simulink library "mfeval_STI_LIB"  (R2017b)
settings: Solver=ode45  StartTime=0.0  StopTime=10.0  RelTol=1e-3
undefined symbols (not defined in the file or in its folder): parameterStruct, userDynamics
libraries: mfeval_LIB x3, mfeval_CPI_LIB x1
settings Model: Creator=MFURLANT  LastModifiedBy=MFURLANT
settings DataIOCC: SaveFormat=StructureWithTime
settings OptimizationCC: LifeSpan=inf
settings DebuggingCC: SFExecutionAtInitializationDiag=none
settings HardwareCC: ProdBitPerSizeT=32  ProdBitPerPtrDiffT=32  ProdWordSize=32  ProdHWDeviceType=Specified
settings CodeAppCC: StateflowObjectComments=on
settings GRTTargetCC: TargetLangStandard=C89/C90 (ANSI)

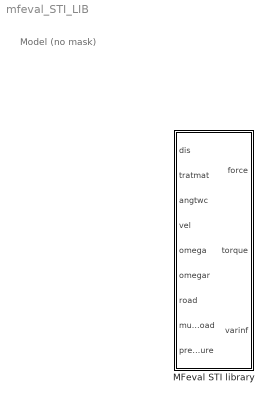
== system mfeval_STI_LIB ==
  note: Model (no mask)
  MFeval STI library : Subsystem

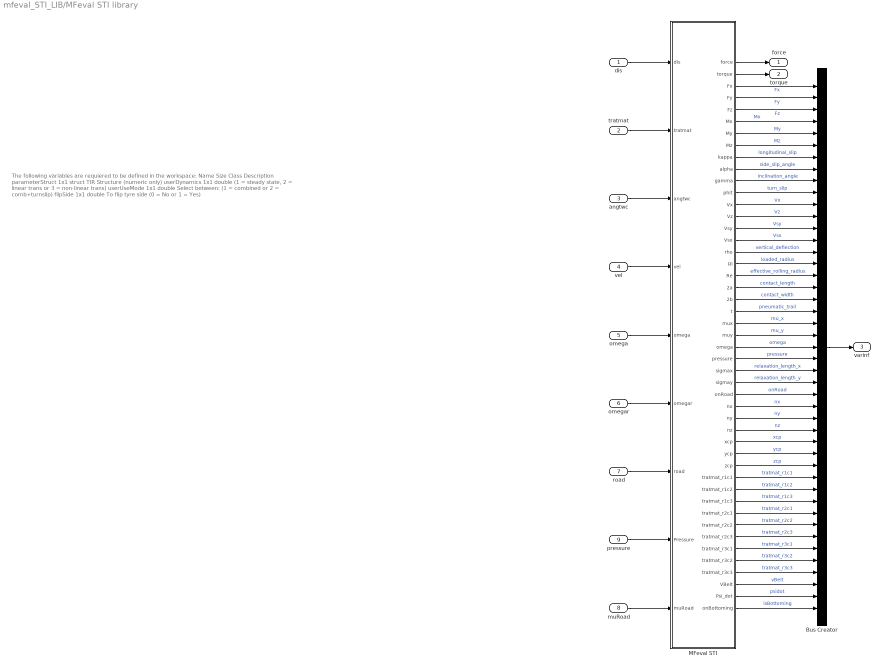
== system mfeval_STI_LIB/MFeval STI library ==
  note: The following variables are requiered to be defined in the workspace:
      |
      | Name
      | Size
      | Class
      | Description
      |
      | parameterStruct
      | 1x1
      | struct
      | TIR Structure (numeric only)
      |
      | userDynamics
      | 1x1
      | double
      | (1 = steady state, 2 = linear trans or 3 = non-linear trans)
      |
      | userUseMode
      | 1x1
      | double
      | Select between: (1 = combined or 2 = comb+turnslip)
      |
      | flipSide
      | 1x1
      | double
      | To flip tyre side (0 = No or 1 = Yes)
  dis : Inport
  tratmat : Inport  Port=2
  angtwc : Inport  Port=3
  vel : Inport  Port=4
  omega : Inport  Port=5
  omegar : Inport  Port=6
  road : Inport  Port=7
  muRoad : Inport  Port=8
  pressure : Inport  Port=9
  Bus Creator : BusCreator  Inputs=45
  MFeval STI : Subsystem
  force : Outport
  torque : Outport  Port=2
  varinf : Outport  Port=3
  wires:
  MFeval STI/7(My) -> Bus Creator/5  "My"
  MFeval STI/17(rho) -> Bus Creator/15  "vertical_deflection"
  MFeval STI/9(kappa) -> Bus Creator/7  "longitudinal_slip"
  MFeval STI/13(Vx) -> Bus Creator/11  "Vx"
  MFeval STI/8(Mz) -> Bus Creator/6  "Mz"
  MFeval STI/14(Vz) -> Bus Creator/12  "Vz"
  MFeval STI/10(alpha) -> Bus Creator/8  "side_slip_angle"
  MFeval STI/16(Vsx) -> Bus Creator/14  "Vsx"
  MFeval STI/1(force) -> force/1
  MFeval STI/2(torque) -> torque/1
  Bus Creator/1 -> varinf/1
  MFeval STI/3(Fx) -> Bus Creator/1  "Fx"
  MFeval STI/4(Fy) -> Bus Creator/2  "Fy"
  MFeval STI/5(Fz) -> Bus Creator/3  "Fz"
  MFeval STI/6(Mx) -> Bus Creator/4  "Mx"
  MFeval STI/19(Re) -> Bus Creator/17  "effective_rolling_radius"
  MFeval STI/15(Vsy) -> Bus Creator/13  "Vsy"
  MFeval STI/18(Rl) -> Bus Creator/16  "loaded_radius"
  MFeval STI/11(gamma) -> Bus Creator/9  "inclination_angle"
  MFeval STI/20(2a) -> Bus Creator/18  "contact_length"
  MFeval STI/27(sigmax) -> Bus Creator/25  "relaxation_length_x"
  MFeval STI/28(sigmay) -> Bus Creator/26  "relaxation_length_y"
  MFeval STI/23(mux) -> Bus Creator/21  "mu_x"
  MFeval STI/22(t) -> Bus Creator/20  "pneumatic_trail"
  MFeval STI/26(pressure) -> Bus Creator/24  "pressure"
  MFeval STI/12(phit) -> Bus Creator/10  "turn_slip"
  MFeval STI/24(muy) -> Bus Creator/22  "mu_y"
  MFeval STI/25("omega ") -> Bus Creator/23  "omega"
  MFeval STI/21(2b) -> Bus Creator/19  "contact_width"
  MFeval STI/29(onRoad) -> Bus Creator/27  "onRoad"
  MFeval STI/30(nx) -> Bus Creator/28  "nx"
  MFeval STI/31(ny) -> Bus Creator/29  "ny"
  MFeval STI/32(nz) -> Bus Creator/30  "nz"
  MFeval STI/33(xcp) -> Bus Creator/31  "xcp"
  MFeval STI/34(ycp) -> Bus Creator/32  "ycp"
  MFeval STI/35(zcp) -> Bus Creator/33  "zcp"
  MFeval STI/36(tratmat_r1c1) -> Bus Creator/34  "tratmat_r1c1"
  MFeval STI/37(tratmat_r1c2) -> Bus Creator/35  "tratmat_r1c2"
  MFeval STI/38(tratmat_r1c3) -> Bus Creator/36  "tratmat_r1c3"
  MFeval STI/39(tratmat_r2c1) -> Bus Creator/37  "tratmat_r2c1"
  MFeval STI/40(tratmat_r2c2) -> Bus Creator/38  "tratmat_r2c2"
  MFeval STI/41(tratmat_r2c3) -> Bus Creator/39  "tratmat_r2c3"
  MFeval STI/42(tratmat_r3c1) -> Bus Creator/40  "tratmat_r3c1"
  MFeval STI/43(tratmat_r3c2) -> Bus Creator/41  "tratmat_r3c2"
  MFeval STI/44(tratmat_r3c3) -> Bus Creator/42  "tratmat_r3c3"
  MFeval STI/45(VBelt) -> Bus Creator/43  "vBelt"
  MFeval STI/46(Psi_dot) -> Bus Creator/44  "psidot"
  muRoad/1 -> MFeval STI/9(muRoad)
  road/1 -> MFeval STI/7(road)
  omegar/1 -> MFeval STI/6(omegar)
  omega/1 -> MFeval STI/5(omega)
  vel/1 -> MFeval STI/4(vel)
  angtwc/1 -> MFeval STI/3(angtwc)
  tratmat/1 -> MFeval STI/2(tratmat)
  dis/1 -> MFeval STI/1(dis)
  pressure/1 -> MFeval STI/8(Pressure)
  MFeval STI/47(onBottoming) -> Bus Creator/45  "isBottoming"

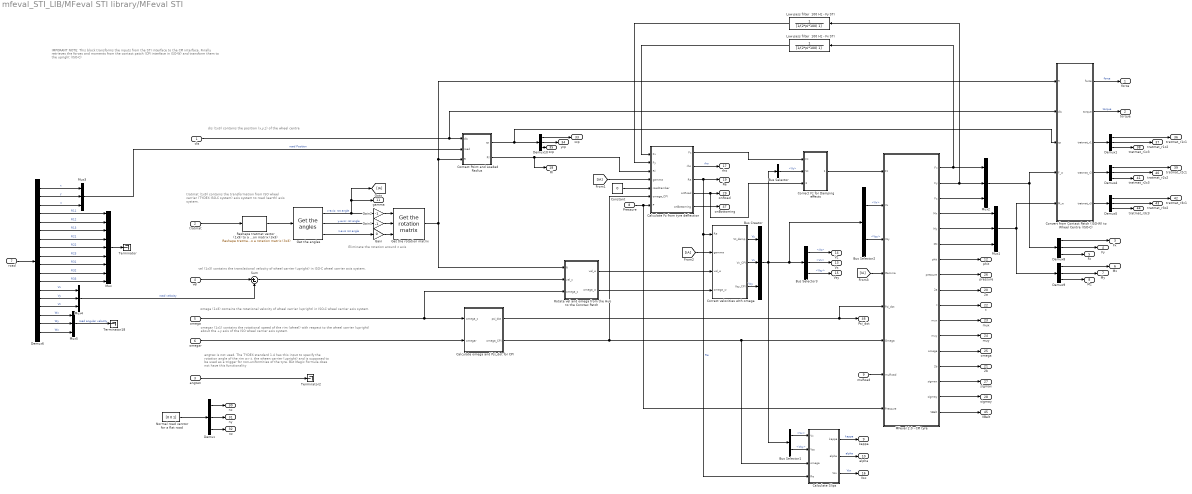
== system mfeval_STI_LIB/MFeval STI library/MFeval STI ==
  note: omegar (1x1) contains the rotational speed of the rim (wheel) with respect to the wheel carrier (upright) about the +y axis of the ISO wheel carrier axis system.
  note: omega (1x3) contains the rotational velocity of wheel carrier (upright) in ISO-C wheel carrier axis system.
  note: tratmat (1x9) contains the transformation from ISO wheel carrier (TYDEX ISO-C system) axis system to road (earth) axis system.
  note: vel (1x3) contains the translational velocity of wheel carrier (upright) in ISO-C wheel carrier axis system.
  note: IMPORANT NOTE:
      |
      | This block transforms the inputs from the STI interface to the CPI interface.
      | Finally retrieves the forces and moments from the contact patch (CPI interface in ISO-W) and transform them to the upright (ISO-C)
  note: angtwc is not used.
      | The TYDEX standard 1.4 has this input to specify the rotation angle of the rim w.r.t. the wheen carrier (upright) and is supposed to be used as a trigger for non-uniformities of the tyre. But Magic Formula does not have this functionality
  note: dis (1x3) contains the position (x,y,z) of the wheel centre
  note: Eliminate the rotation around z axis
  dis : Inport
  tratmat : Inport  Port=2
  angtwc : Inport  Port=3
  vel : Inport  Port=4
  omega : Inport  Port=5
  omegar : Inport  Port=6
  road : Inport  Port=7
  Pressure : Inport  Port=8
  muRoad : Inport  Port=9
  Bus Creator : BusCreator  Inputs=3
  Bus Selector : BusSelector  OutputSignals=Vz
  Bus Selector1 : BusSelector  OutputSignals=Vx,Vsy
  Bus Selector2 : BusSelector  OutputSignals=Vx,Vsy
  Bus Selector3 : BusSelector  OutputSignals=Vz,Vx,Vsy
  Calculate Fz from tyre deflection : MATLAB Function  TreatAsAtomicUnit=on
  Calculate Slips : MATLAB Function  TreatAsAtomicUnit=on
  Calculate omega and Psi_dot for CPI : Subsystem
  Constant : Constant  Value=0
  Contact Point and Loaded Radius : MATLAB Function  TreatAsAtomicUnit=on
  Convert from Contact Patch (ISO-W) to Wheel Centre (ISO-C) : MATLAB Function  TreatAsAtomicUnit=on
  Correct Fz for Damping effects : Subsystem
  Correct velocities with omega : Subsystem
  Demux{,1,4..5,8..10} (7 alike) : Demux  Outputs=3
  Demux6 : Demux  Outputs=18
  Gain : Gain  Gain=0
  Gain1 : Gain  Gain=-1
  Gain2 : Gain  Gain=-1
  Get the angles : mfeval_LIB/Get the angles
      settings: SourceProductName=MFeval Library
  Get the rotation matrix : mfeval_LIB/Get the rotation matrix
      settings: SourceProductName=MFeval Library
  Low pass filter  100 Hz - Fx STI : TransferFcn  Denominator=[1/(2*pi*100) 1]
  Low pass filter  100 Hz - Fy STI : TransferFcn  Denominator=[1/(2*pi*100) 1]
  MFeval 2.0 - CPI tyre : Subsystem
  Mux : Mux  Inputs=9
  Mux{1..5} (5 alike) : Mux  Inputs=3
  Normal road verctor for a flat road : Constant  Value=[0 0 1]
  Reshape tratmat vector (1x9) to a rotation matrix (3x3) : mfeval_LIB/Reshape tratmat vector (1x9)  to a rotation matrix (3x3)
      settings: SourceProductName=MFeval Library
  Rotate vel and omega from the Hub to the Conctac Patch : Subsystem
  Sum : Sum  Inputs=|+-
  Terminator : Terminator
  Terminator18 : Terminator
  Terminator2 : Terminator
  force : Outport
  torque : Outport  Port=2
  Fx : Outport  Port=3
  Fy : Outport  Port=4
  Fz : Outport  Port=5
  Mx : Outport  Port=6
  My : Outport  Port=7
  Mz : Outport  Port=8
  kappa : Outport  Port=9
  alpha : Outport  Port=10
  gamma : Outport  Port=11
  phit : Outport  Port=12
  Vx : Outport  Port=13
  Vz : Outport  Port=14
  Vsy : Outport  Port=15
  Vsx : Outport  Port=16
  rho : Outport  Port=17
  Rl : Outport  Port=18
  Re : Outport  Port=19
  2a : Outport  Port=20
  2b : Outport  Port=21
  t : Outport  Port=22
  mux : Outport  Port=23
  muy : Outport  Port=24
  "omega " : Outport  Port=25
  pressure : Outport  Port=26
  sigmax : Outport  Port=27
  sigmay : Outport  Port=28
  onRoad : Outport  Port=29
  nx : Outport  Port=30
  ny : Outport  Port=31
  nz : Outport  Port=32
  xcp : Outport  Port=33
  ycp : Outport  Port=34
  zcp : Outport  Port=35
  tratmat_r1c1 : Outport  Port=36
  tratmat_r1c2 : Outport  Port=37
  tratmat_r1c3 : Outport  Port=38
  tratmat_r2c1 : Outport  Port=39
  tratmat_r2c2 : Outport  Port=40
  tratmat_r2c3 : Outport  Port=41
  tratmat_r3c1 : Outport  Port=42
  tratmat_r3c2 : Outport  Port=43
  tratmat_r3c3 : Outport  Port=44
  VBelt : Outport  Port=45
  Psi_dot : Outport  Port=46
  onBottoming : Outport  Port=47
  wires:
  Contact Point and Loaded Radius/2(Rl) -> Rl/1, Calculate Fz from tyre deflection/3(Rl)
  angtwc/1 -> Terminator2/1
  MFeval 2.0 - CPI tyre/1(Fx) -> Low pass filter  100 Hz - Fx STI/1, Mux2/1
  MFeval 2.0 - CPI tyre/2(Fy) -> Low pass filter  100 Hz - Fy STI/1, Mux2/2
  tratmat/1 -> Reshape tratmat vector (1x9) to a rotation matrix (3x3)/1
  MFeval 2.0 - CPI tyre/4(Mx) -> Mux1/1
  MFeval 2.0 - CPI tyre/5(My) -> Mux1/2
  Mux1/1 -> Convert from Contact Patch (ISO-W) to Wheel Centre (ISO-C)/5(M_w), Demux9/1
  Mux2/1 -> Convert from Contact Patch (ISO-W) to Wheel Centre (ISO-C)/4(F_w), Demux8/1
  MFeval 2.0 - CPI tyre/3("Fz ") -> Mux2/3
  Get the angles/3 -> Gain/1  "z-axis rot angle"
  Get the angles/2 -> Gain1/1  "y-axis: rot angle"
  Convert from Contact Patch (ISO-W) to Wheel Centre (ISO-C)/1(force) -> force/1  "force"
  Convert from Contact Patch (ISO-W) to Wheel Centre (ISO-C)/2(torque) -> torque/1  "torque"
  omegar/1 -> Calculate omega and Psi_dot for CPI/2(omegar)
  Calculate Fz from tyre deflection/2(rho) -> rho/1  "rho"
  Calculate omega and Psi_dot for CPI/2(omega_CPI) -> Calculate Fz from tyre deflection/6(omega_CPI), MFeval 2.0 - CPI tyre/6(Omega), Calculate Slips/3(omega)
  Sum/1 -> Rotate vel and omega from the Hub to the Conctac Patch/2(vel_c)
  Calculate Fz from tyre deflection/1(Fz) -> Correct Fz for Damping effects/1(Fz)
  MFeval 2.0 - CPI tyre/6(Mz) -> Mux1/3
  MFeval 2.0 - CPI tyre/7(phit) -> phit/1
  MFeval 2.0 - CPI tyre/8(pressure) -> pressure/1
  MFeval 2.0 - CPI tyre/9(2a) -> 2a/1
  MFeval 2.0 - CPI tyre/10(t) -> t/1
  MFeval 2.0 - CPI tyre/11(mux) -> mux/1
  MFeval 2.0 - CPI tyre/12(muy) -> muy/1
  MFeval 2.0 - CPI tyre/13(omega) -> "omega "/1
  MFeval 2.0 - CPI tyre/14(2b) -> 2b/1
  MFeval 2.0 - CPI tyre/15(sigmax) -> sigmax/1
  MFeval 2.0 - CPI tyre/16(sigmay) -> sigmay/1
  Rotate vel and omega from the Hub to the Conctac Patch/1(vel_w) -> Correct velocities with omega/3(vel_w)
  Rotate vel and omega from the Hub to the Conctac Patch/2(omega_w) -> Correct velocities with omega/4(omega_w)
  Calculate Slips/1(kappa) -> kappa/1  "kappa"
  Calculate Slips/2(alpha) -> alpha/1  "alpha"
  Calculate Slips/3(Vsx) -> Vsx/1  "Vsx"
  Calculate Fz from tyre deflection/3(Re) -> Calculate Slips/4(Re), Correct velocities with omega/1(Re), Re/1  "Re"
  Correct velocities with omega/1(Vz_damp) -> Bus Creator/1  "Vz"
  Correct velocities with omega/2(Vx_CPI) -> Bus Creator/2  "Vx"
  Correct velocities with omega/3(Vsy_CPI) -> Bus Creator/3  "Vsy"
  Bus Creator/1 -> Bus Selector1/1, Bus Selector2/1, Bus Selector3/1, Bus Selector/1
  Bus Selector/1 -> Correct Fz for Damping effects/2(Vz)  "<Vz>"
  Bus Selector1/1 -> Calculate Slips/1(Vx)  "<Vx>"
  Bus Selector1/2 -> Calculate Slips/2(Vsy)  "<Vsy>"
  Bus Selector2/1 -> MFeval 2.0 - CPI tyre/2(Vx)  "<Vx>"
  Bus Selector2/2 -> MFeval 2.0 - CPI tyre/3(Vsy)  "<Vsy>"
  Bus Selector3/3 -> Vsy/1  "<Vsy>"
  Bus Selector3/2 -> Vx/1  "<Vx>"
  Bus Selector3/1 -> Vz/1  "<Vz>"
  Low pass filter  100 Hz - Fy STI/1 -> Calculate Fz from tyre deflection/2(Fy)
  Low pass filter  100 Hz - Fx STI/1 -> Calculate Fz from tyre deflection/1(Fx)
  Demux10/1 -> xcp/1
  Demux10/2 -> ycp/1
  Demux10/3 -> zcp/1
  Convert from Contact Patch (ISO-W) to Wheel Centre (ISO-C)/3(tratmat_r1) -> Demux1/1
  Convert from Contact Patch (ISO-W) to Wheel Centre (ISO-C)/4(tratmat_r2) -> Demux4/1
  Convert from Contact Patch (ISO-W) to Wheel Centre (ISO-C)/5(tratmat_r3) -> Demux5/1
  Demux1/1 -> tratmat_r1c1/1
  Demux1/2 -> tratmat_r1c2/1
  Demux1/3 -> tratmat_r1c3/1
  Demux4/1 -> tratmat_r2c1/1
  Demux4/2 -> tratmat_r2c2/1
  Demux4/3 -> tratmat_r2c3/1
  Demux5/1 -> tratmat_r3c1/1
  Demux5/2 -> tratmat_r3c2/1
  Demux5/3 -> tratmat_r3c3/1
  MFeval 2.0 - CPI tyre/17(VBelt) -> VBelt/1
  road/1 -> Demux6/1
  Demux6/1 -> Mux3/1  "x"
  Demux6/2 -> Mux3/2  "y"
  Demux6/3 -> Mux3/3  "z"
  Demux6/4 -> Mux/1  "R11"
  Demux6/5 -> Mux/2  "R12"
  Demux6/6 -> Mux/3  "R13"
  Demux6/7 -> Mux/4  "R21"
  Demux6/8 -> Mux/5  "R22"
  Demux6/9 -> Mux/6  "R23"
  Demux6/10 -> Mux/7  "R31"
  Demux6/11 -> Mux/8  "R32"
  Demux6/12 -> Mux/9  "R33"
  Demux6/13 -> Mux4/1  "Vx"
  Demux6/14 -> Mux4/2  "Vy"
  Demux6/15 -> Mux4/3  "Vz"
  Demux6/16 -> Mux5/1  "Wx"
  Demux6/17 -> Mux5/2  "Wy"
  Demux6/18 -> Mux5/3  "Wz"
  Mux3/1 -> Contact Point and Loaded Radius/2(road)  "road Position"
  Mux4/1 -> Sum/2  "road velocity"
  Get the angles/1 -> gamma/1, [IA], Gain2/1  "x-axis: rot angle"
  Demux8/1 -> Fx/1
  Demux8/2 -> Fy/1
  Demux8/3 -> Fz/1
  Demux9/1 -> Mx/1
  Demux9/2 -> My/1
  Demux9/3 -> Mz/1
  Demux/2 -> ny/1
  Demux/3 -> nz/1
  Demux/1 -> nx/1
  Normal road verctor for a flat road/1 -> Demux/1
  Constant/1 -> Calculate Fz from tyre deflection/5(roadCamber)
  dis/1 -> Convert from Contact Patch (ISO-W) to Wheel Centre (ISO-C)/2(dis), Contact Point and Loaded Radius/1(dis)
  Mux5/1 -> Terminator18/1  "road angular velocity"
  vel/1 -> Sum/1
  muRoad/1 -> MFeval 2.0 - CPI tyre/7(muRoad)
  Get the rotation matrix/1 -> Convert from Contact Patch (ISO-W) to Wheel Centre (ISO-C)/1(R), Contact Point and Loaded Radius/3(R), Rotate vel and omega from the Hub to the Conctac Patch/1(R)
  [IA] -> Calculate Fz from tyre deflection/4(gamma)
  [IA] -> Correct velocities with omega/2(gamma)
  [IA] -> MFeval 2.0 - CPI tyre/4(Gamma)
  Calculate Fz from tyre deflection/4(onRoad) -> Correct Fz for Damping effects/3(onRoad), onRoad/1
  Correct Fz for Damping effects/1(Fz_CPI) -> MFeval 2.0 - CPI tyre/1(Fz)
  Pressure/1 -> MFeval 2.0 - CPI tyre/8(Pressure), Calculate Fz from tyre deflection/7(P)
  omega/1 -> Rotate vel and omega from the Hub to the Conctac Patch/3(omega_c), Calculate omega and Psi_dot for CPI/1(omega_c)
  Calculate omega and Psi_dot for CPI/1(psi_dot) -> MFeval 2.0 - CPI tyre/5(Psi_dot), Psi_dot/1
  Calculate Fz from tyre deflection/5(onBottoming) -> onBottoming/1
  Contact Point and Loaded Radius/1(cp) -> Convert from Contact Patch (ISO-W) to Wheel Centre (ISO-C)/3(cp), Demux10/1
  Mux/1 -> Terminator/1
  Gain/1 -> Get the rotation matrix/3
  Reshape tratmat vector (1x9) to a rotation matrix (3x3)/1 -> Get the angles/1
  Gain1/1 -> Get the rotation matrix/2
  Gain2/1 -> Get the rotation matrix/1

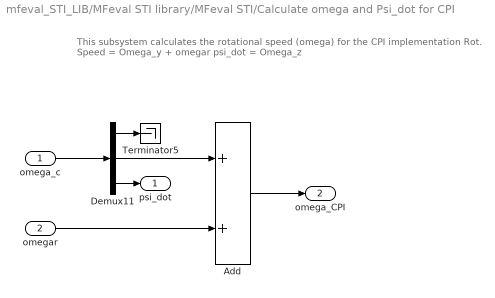
== system mfeval_STI_LIB/MFeval STI library/MFeval STI/Calculate omega and Psi_dot for CPI ==
  note: This subsystem calculates the rotational speed (omega) for the CPI implementation
      |
      | Rot. Speed = Omega_y + omegar
      | psi_dot = Omega_z
  omega_c : Inport
  omegar : Inport  Port=2
  Add : Sum
  Demux11 : Demux  Outputs=3
  Terminator5 : Terminator
  psi_dot : Outport
  omega_CPI : Outport  Port=2
  wires:
  Add/1 -> omega_CPI/1
  omega_c/1 -> Demux11/1
  omegar/1 -> Add/2
  Demux11/1 -> Terminator5/1
  Demux11/3 -> psi_dot/1
  Demux11/2 -> Add/1

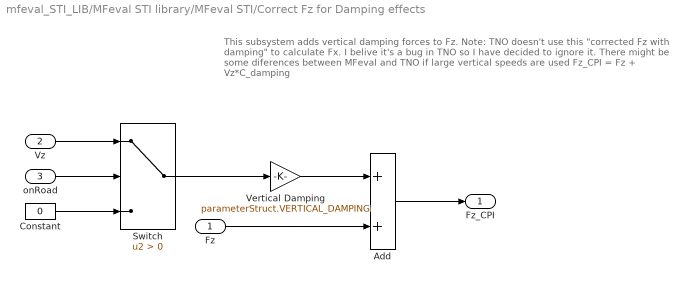
== system mfeval_STI_LIB/MFeval STI library/MFeval STI/Correct Fz for Damping effects ==
  note: This subsystem adds vertical damping forces to Fz.
      |
      | Note: TNO doesn't use this "corrected Fz with damping" to calculate Fx.
      | I belive it's a bug in TNO so I have decided to ignore it.
      | There might be some diferences between MFeval and TNO if large vertical speeds are used
      |
      |
      | Fz_CPI = Fz + Vz*C_damping
  Fz : Inport
  Vz : Inport  Port=2
  onRoad : Inport  Port=3
  Add : Sum
  Constant : Constant  Value=0
  Switch : Switch  Criteria=u2 > Threshold
  Vertical Damping : Gain  Gain=parameterStruct.VERTICAL_DAMPING
  Fz_CPI : Outport
  wires:
  Fz/1 -> Add/2
  Add/1 -> Fz_CPI/1
  Vz/1 -> Switch/1
  Vertical Damping/1 -> Add/1
  onRoad/1 -> Switch/2
  Constant/1 -> Switch/3
  Switch/1 -> Vertical Damping/1

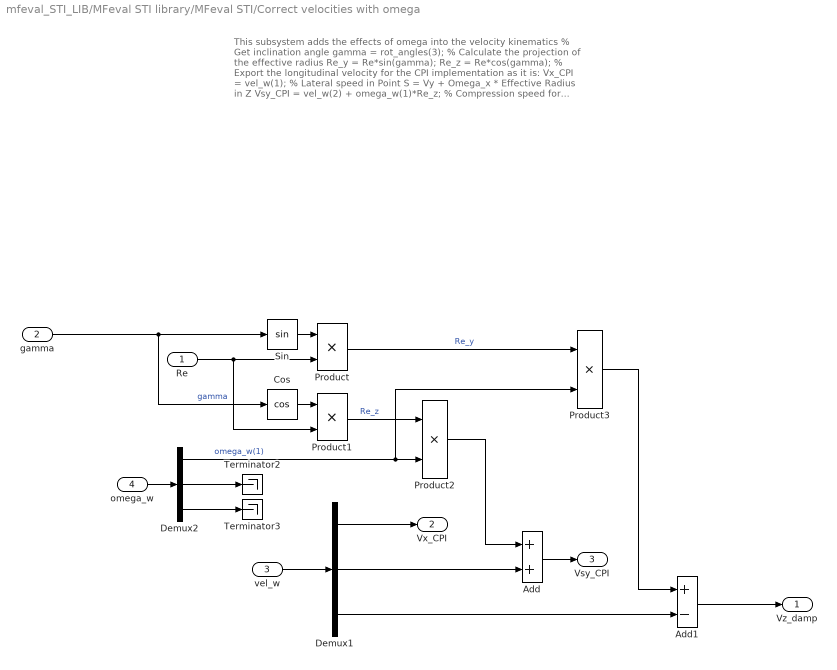
== system mfeval_STI_LIB/MFeval STI library/MFeval STI/Correct velocities with omega ==
  note: This subsystem adds the effects of omega into the velocity kinematics
      |
      | % Get inclination angle
      | gamma = rot_angles(3);
      |
      | % Calculate the projection of the effective radius
      | Re_y = Re*sin(gamma);
      | Re_z = Re*cos(gamma);
      |
      | % Export the longitudinal velocity for the CPI implementation as it is:
      | Vx_CPI = vel_w(1);
      |
      | % Lateral speed in Point S = Vy + Omega_x * Effective Radius in Z
      | Vsy_CPI = vel_w(2) + omega_w(1)*Re_z;
      |
      | % Compression speed for damping effects:
      | Vz_damp = vel_w(3) + omega_w(1)*Re_y;
  Re : Inport
  gamma : Inport  Port=2
  vel_w : Inport  Port=3
  omega_w : Inport  Port=4
  Add : Sum
  Add1 : Sum  Inputs=+-
  Cos : Trigonometry  Operator=cos
  Demux1 : Demux  Outputs=3
  Demux2 : Demux  Outputs=3
  Product{,1..3} (4 alike) : Product
  Sin : Trigonometry
  Terminator2 : Terminator
  Terminator3 : Terminator
  Vz_damp : Outport
  Vx_CPI : Outport  Port=2
  Vsy_CPI : Outport  Port=3
  wires:
  gamma/1 -> Sin/1, Cos/1  "gamma"
  Sin/1 -> Product/1
  Re/1 -> Product1/2, Product/2
  Cos/1 -> Product1/1
  Product/1 -> Product3/1  "Re_y"
  Product1/1 -> Product2/1  "Re_z"
  vel_w/1 -> Demux1/1
  Demux1/1 -> Vx_CPI/1
  Demux1/2 -> Add/2
  omega_w/1 -> Demux2/1
  Demux2/3 -> Terminator3/1
  Demux2/2 -> Terminator2/1
  Demux2/1 -> Product3/2, Product2/2  "omega_w(1)"
  Product2/1 -> Add/1
  Add/1 -> Vsy_CPI/1
  Product3/1 -> Add1/1
  Demux1/3 -> Add1/2
  Add1/1 -> Vz_damp/1

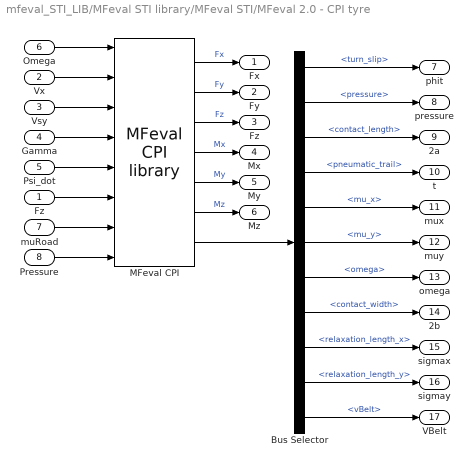
== system mfeval_STI_LIB/MFeval STI library/MFeval STI/MFeval 2.0 - CPI tyre ==
  Fz : Inport
  Vx : Inport  Port=2
  Vsy : Inport  Port=3
  Gamma : Inport  Port=4
  Psi_dot : Inport  Port=5
  Omega : Inport  Port=6
  muRoad : Inport  Port=7
  Pressure : Inport  Port=8
  Bus Selector : BusSelector  OutputSignals=turn_slip,pressure,contact_length,pneumatic_trail,mu_x,mu_y,omega,contact_width,relaxation_length_x,relaxation_length_y,vBelt
  MFeval CPI : mfeval_CPI_LIB/MFeval CPI library
  Fx : Outport
  Fy : Outport  Port=2
  "Fz " : Outport  Port=3
  Mx : Outport  Port=4
  My : Outport  Port=5
  Mz : Outport  Port=6
  phit : Outport  Port=7
  pressure : Outport  Port=8
  2a : Outport  Port=9
  t : Outport  Port=10
  mux : Outport  Port=11
  muy : Outport  Port=12
  omega : Outport  Port=13
  2b : Outport  Port=14
  sigmax : Outport  Port=15
  sigmay : Outport  Port=16
  VBelt : Outport  Port=17
  wires:
  Omega/1 -> MFeval CPI/1
  Vx/1 -> MFeval CPI/2
  Vsy/1 -> MFeval CPI/3
  Gamma/1 -> MFeval CPI/4
  Psi_dot/1 -> MFeval CPI/5
  MFeval CPI/1 -> Fx/1  "Fx"
  MFeval CPI/2 -> Fy/1  "Fy"
  MFeval CPI/3 -> "Fz "/1  "Fz"
  MFeval CPI/4 -> Mx/1  "Mx"
  MFeval CPI/5 -> My/1  "My"
  MFeval CPI/6 -> Mz/1  "Mz"
  Bus Selector/2 -> pressure/1  "<pressure>"
  Bus Selector/1 -> phit/1  "<turn_slip>"
  Bus Selector/7 -> omega/1  "<omega>"
  Bus Selector/8 -> 2b/1  "<contact_width>"
  Bus Selector/3 -> 2a/1  "<contact_length>"
  Bus Selector/4 -> t/1  "<pneumatic_trail>"
  Bus Selector/5 -> mux/1  "<mu_x>"
  Bus Selector/6 -> muy/1  "<mu_y>"
  Bus Selector/9 -> sigmax/1  "<relaxation_length_x>"
  Bus Selector/10 -> sigmay/1  "<relaxation_length_y>"
  Bus Selector/11 -> VBelt/1  "<vBelt>"
  Fz/1 -> MFeval CPI/6
  MFeval CPI/7 -> Bus Selector/1
  muRoad/1 -> MFeval CPI/7
  Pressure/1 -> MFeval CPI/8

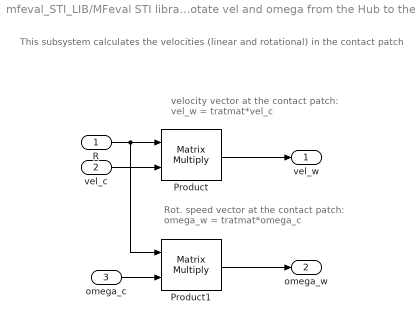
== system mfeval_STI_LIB/MFeval STI library/MFeval STI/Rotate vel and omega from the Hub to the Conctac Patch ==
  note: Rot. speed vector at the contact patch:
      | omega_w = tratmat*omega_c
  note: velocity vector at the contact patch:
      | vel_w = tratmat*vel_c
  note: This subsystem calculates the velocities (linear and rotational) in the contact patch
  R : Inport
  vel_c : Inport  Port=2
  omega_c : Inport  Port=3
  Product : Product  Multiplication=Matrix(*)
  Product1 : Product  Multiplication=Matrix(*)
  vel_w : Outport
  omega_w : Outport  Port=2
  wires:
  R/1 -> Product1/1, Product/1
  Product/1 -> vel_w/1
  omega_c/1 -> Product1/2
  Product1/1 -> omega_w/1
  vel_c/1 -> Product/2

== matlab function mfeval_STI_LIB/MFeval STI library/MFeval STI/Contact Point and Loaded Radius ==
  data: dis input; road input; cp output; R input; Rl output
function [cp, Rl] = fcn(dis, road, R)

% Pre-allocate
cp = [0; 0; 0];

% Normal vectors
nEarth = [0;0;1];
nCAxis = R*nEarth;

% Straight line equation
%   x = dis(1)+nCAxis(1)*t
%   y = dis(2)+nCAxis(2)*t
%   z = dis(3)+nCAxis(3)*t

% Flat road plane equation
%   z = road(3)

% Intersection between a straight line and a plane
t = (road(3)- dis(3))/nCAxis(3);
cp(1) = dis(1)+nCAxis(1)*t;
cp(2) = dis(2)+nCAxis(2)*t;
cp(3) = dis(3)+nCAxis(3)*t;

% Calculate the loaded radius
Rl = sqrt((dis(1)-cp(1))^2+(dis(2)-cp(2))^2+(dis(3)-cp(3))^2);

== matlab function mfeval_STI_LIB/MFeval STI library/MFeval STI/Calculate Slips ==
  data: parameterStruct parameter; Vx input; Vsy input; omega input; Re input; kappa output; alpha output; Vsx output
function [kappa, alpha, Vsx]  = fcn(parameterStruct, Vx, Vsy, omega, Re)
%#codegen

% This function calculates the slip inputs without damping effects. 
% Note that these slip inputs are not used in the CPI calculations. 
% This is how TNO has implemented the calculations, so here we are
% doing the same...


% Longitudinal slip velocity
Vsx = Vx - Re.*omega; % [Eqn (2.3) Page 64 - Book]

% Check if is low speed
isLowSpeed = abs(Vx) < parameterStruct.VXLOW;

if isLowSpeed
    % Avoid sign(0) = 0
    signVx = sign(Vx);
    signVx(signVx == 0) = 1;
   
    % Low speed Slip Ratio Calculation
    kappa = -(Vsx) * signVx;
else
    % Slip Ratio Calculation
    kappa = -(Vsx./Vx); % [Eqn (2.4) Page 64 - Book]
end

if isnan(kappa)
    kappa = 0;
end

% Slip Angle
alpha = atan(Vsy./abs(Vx)); % [Eqn (2.9) Page 67 - Book]

% Important Note:
% Due to the ISO sign convention, equation 2.9 does not need a
% negative sign. The pacejka book is written in adapted SAE.

if isnan(alpha)
    alpha = 0;
end

== matlab function mfeval_STI_LIB/MFeval STI library/MFeval STI/Calculate Fz from tyre deflection ==
  data: parameterStruct parameter; Fx input; Fy input; Rl input; gamma input; roadCamber input; Fz output; omega_CPI input; P input; rho output; Re output; userDynamics parameter; onRoad output; onBottoming output
function [Fz, rho, Re, onRoad, onBottoming] = fcn(parameterStruct, Fx, Fy, Rl, gamma, roadCamber, omega_CPI, P, userDynamics)
%#codegen


% This function calculates the Fz from the tyre deflection

%[MODEL]
Vo      = parameterStruct.LONGVL               ; %Nominal speed
pio     = parameterStruct.NOMPRES              ; %Reference pressure

%[VERTICAL]
Fzo     = parameterStruct.FNOMIN         		; %Nominal wheel load
Cz0     = parameterStruct.VERTICAL_STIFFNESS	; %Tyre vertical stiffness
Q_RE0	= parameterStruct.Q_RE0       			; %Ratio of free tyre radius with nominal tyre radius
Q_V1	= parameterStruct.Q_V1  				; %Tyre radius increase with speed
Q_V2	= parameterStruct.Q_V2    				; %Vertical stiffness increase with speed
Q_FZ2	= parameterStruct.Q_FZ2      			; %Quadratic term in load vs. deflection
PFZ1	= parameterStruct.PFZ1    				; %Pressure effect on vertical stiffness
Q_FCX    = parameterStruct.Q_FCX;
Q_FCY    = parameterStruct.Q_FCY;

BREFF   = parameterStruct.BREFF      			; %Low load stiffness effective rolling radius
DREFF	= parameterStruct.DREFF     			; %Peak value of effective rolling radius
FREFF	= parameterStruct.FREFF    			; %High load stiffness effective rolling radius

BOTTOM_OFFST = parameterStruct.BOTTOM_OFFST    ; %Distance to rim when bottoming starts to occur
BOTTOM_STIFF = parameterStruct.BOTTOM_STIFF    ; %Vertical stiffness of bottomed tyre

%[DIMENSION]
Ro          = parameterStruct.UNLOADED_RADIUS      ; %Free tyre radius
RIM_RADIUS  = parameterStruct.RIM_RADIUS          ; %Nominal rim radius

% Normalized change in inflation pressure
dpi = (P - pio)./pio; % [Eqn (4.E2b) Page 177 - Book]

% Free-spinning radius
Romega = Ro .* (Q_RE0 + Q_V1.*((omega_CPI.*Ro)./Vo).^2); % [Eqn (1) Page 2 - Paper] - Centrifugal growth of the free tyre radius

% Nominal stiffness (pressure corrected)
Cz = Cz0 .* (1 + PFZ1.*dpi); % [Eqn (5) Page 2 - Paper] - Vertical stiffness adapted for tyre inflation pressure

% Tyre deflection
rhoz0 = max((Romega-Rl),0);

rho = rhoz0/cos(-roadCamber);

% Model parameters as QFZ1 that normally aren't present in the TIR files
Q_FZ1 = sqrt((Cz0.*Ro./Fzo).^2 - 4.* Q_FZ2); % Rearranging [Eqn (4) Page 2 - Paper]

if userDynamics == 1
    % Calculate Fz without external effects
    Fz = (1 + Q_V2*(Ro/Vo)*abs(omega_CPI))*(Q_FZ1*(rho/Ro)+ Q_FZ2*(rho/Ro)^2)*(1+PFZ1*dpi)*Fzo; % [Eqn (3) Page 2 - Paper]
else
    if parameterStruct.FITTYP == 61
        % Calculate Fz with MF6.1 equations
        Fz = (1 + Q_V2*(Ro/Vo)*abs(omega_CPI)-(Q_FCX*Fx/Fzo)^2-(Q_FCY*Fy/Fzo)^2)*(Q_FZ1*(rho/Ro)+ Q_FZ2*(rho/Ro)^2)*(1+PFZ1*dpi)*Fzo; % [Eqn (3) Page 2 - Paper]
    else
        solver = mfeval.Solver;
        [Fz, rho] = solver.calculateFz62(parameterStruct, gamma, omega_CPI, Romega, dpi, Rl, Fx, Fy);
    end
end

% Variable to determine if there is wheel lift
if rho == 0
    onRoad = 0;
else
    onRoad = 1;
end

% Bottoming model:
Fz_btm = BOTTOM_STIFF * (RIM_RADIUS+BOTTOM_OFFST-Rl); %Equation on page 22 of the TNO Equation Manual (Bottoming model)

if Fz_btm>Fz
    Fz = Fz_btm;
    onBottoming = 1;
else
    onBottoming = 0;
end

% Effective Rolling Radius
Re = Romega -(Fzo./Cz) .* ( DREFF .*atan( BREFF.*(Fz./Fzo)) + FREFF.*(Fz./Fzo)); % [Eqn (7) Page 2 - Paper]

== matlab function mfeval_STI_LIB/MFeval STI library/MFeval STI/Convert from Contact Patch (ISO-W) to Wheel Centre (ISO-C) ==
  data: R input; dis input; cp input; force output; torque output; F_w input; M_w input; tratmat_r1 output; tratmat_r2 output; tratmat_r3 output
function [force, torque, tratmat_r1, tratmat_r2,tratmat_r3]= fcn(R, dis, cp, F_w, M_w)
%#codegen

% This function rotates and translates forces and moments from the 
% contact patch to the wheel centre

% Vector from the wheel center (dis) to the contact point (cp)
DisCp = cp-dis;

% Equivalent moments in the wheel center
M_c = M_w + cross(DisCp, F_w);

% Rotation of forces and moments:
force = R'*F_w;
torque = R'*M_c;

% Export transformation matrix rows
tratmat_r1 = R(1,:)';
tratmat_r2 = R(2,:)';
tratmat_r3 = R(3,:)';
